simulink model "power_svc_1t_1phase_d"  (R2019a)
settings: Solver=VariableStepAuto  StartTime=0.0  StopTime=0.6  FixedStep=Ts  MaxStep=Ts  RelTol=1e-4  AbsTol=1e-4
PreLoadFcn:
  | Ts=50e-6;
libraries: powerlib x9
settings Model: ExtModeTrigMode=oneshot  ExtModeArmWhenConnect=off  ExtModeAutoUpdateStatusClock=off  Creator=MathWorks  LastModifiedBy=Thiago
settings SolverCC: AutoScaleAbsTol=off  ShapePreserveControl=EnableAll  ZeroCrossControl=EnableAll
settings DataIOCC: SaveFormat=StructureWithTime  SignalLoggingSaveFormat=ModelDataLogs  SaveOutput=off  SignalLogging=off  DSMLogging=off  SaveTime=off  ReturnWorkspaceOutputs=off  SignalLoggingName=sigsOut
settings OptimizationCC: BooleanDataType=off  ExpressionDepthLimit=2147483647  InitFltsAndDblsToZero=on  EfficientMapNaN2IntZero=off  LifeSpan=inf
settings DebuggingCC: UnderspecifiedInitializationDetection=Classic  MergeDetectMultiDrivingBlocksExec=none  CheckExecutionContextPreStartOutputMsg=on  CheckExecutionContextRuntimeOutputMsg=on  SignalResolutionControl=TryResolveAllWithWarning  MultiTaskDSMMsg=warning  MultiTaskCondExecSysMsg=none  FcnCallInpInsideContextMsg=warning  AllowSymbolicDim=off  StateNameClashWarn=warning  SFUnexpectedBacktrackingDiag=warning  SFNoUnconditionalDefaultTransitionDiag=warning  SFExecutionAtInitializationDiag=none  ArithmeticOperatorsInVariantConditions=warning
settings HardwareCC: ProdBitPerPointer=32  ProdBitPerSizeT=32  ProdBitPerPtrDiffT=32  ProdLargestAtomicFloat=None  ProdIntDivRoundTo=Undefined  ProdEndianess=Unspecified  ProdWordSize=32  ProdHWDeviceType=32-bit Generic  TargetUnknown=on
settings ModelReferenceCC: PropagateSignalLabelsOutOfModel=off
settings SFSimCC: SimUseLocalCustomCode=off
settings RTWCC: RTWUseLocalCustomCode=off
settings CodeAppCC: StateflowObjectComments=on
settings GRTTargetCC: TargetLangStandard=C89/C90 (ANSI)  CombineOutputUpdateFcns=off  GRTInterface=on
settings ConfigComp: CovMetricSettings=dw  CovSaveCumulativeToWorkspaceVar=on  CovSaveSingleToWorkspaceVar=on  CovExternalEMLEnable=off  CovSFcnEnable=off
settings SimscapeCC: SimscapeNormalizeSystem=off

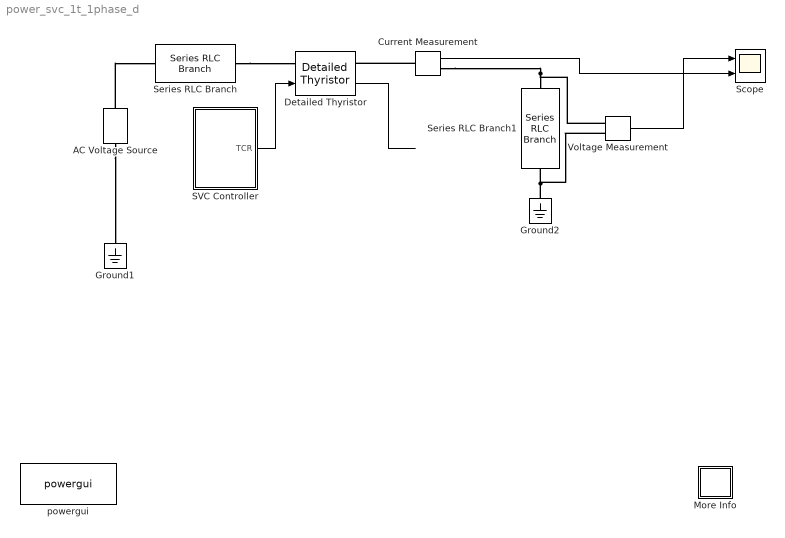
== system power_svc_1t_1phase_d ==
  AC Voltage Source : powerlib/Electrical Sources/AC Voltage Source  Amplitude=179.6  Phase=0  Frequency=60  SampleTime=0  Measurements=Voltage  BusType=swing  Pref=10e3  Qref=0  Qmin=-inf  Qmax=+inf
  Current Measurement : powerlib/Measurements/Current Measurement  PhasorSimulation=off  OutputType=Complex  PSBequivalent=0
  Detailed Thyristor : powerlib/Power Electronics/Detailed Thyristor  Ron=0.001  Lon=1e-3  Vf=0.8  IL=0.1  Tq=100e-6  IC=0.01  Rs=500  Cs=250e-9  Measurements=on
      settings: SourceProductBaseCode=PS
  Ground1 : powerlib/Elements/Ground  LConnTagsString=a
  Ground2 : powerlib/Elements/Ground  LConnTagsString=a
  More Info : Subsystem
      settings: OpenFcn=showdemo(bdroot(gcb))
      mask Display: disp('?')
  SVC Controller : Subsystem  mask(SVC Controller){OpMode=Voltage regulation, Vref=1.0, KpKi=[0 800], Xs=0.01, Bmin_max=[-1.04  3.23], Bref=2.5, Ts=Ts}
      mask prompts: OpMode "Operation mode"; Vref "Reference voltage (pu):"; KpKi "Regulator gains [ Kp  Ki ]:"; Xs "Droop (pu/100MVA):"; Bmin_max "Min. and max. primary susceptances [ Bind Bcap] (pu/100MVA):"; Bref "Susceptance Bref (pu/100MVA) (Var control mode):"; Ts "Sample time (s):"
      mask help:
      | This block implements a controller for a Static Var Compensator (SVC) consisting of one thyristor-controlled reactor bank (TCR) and three thyristor-switched capacitor banks (TSCs). Outputs TCR, TSC1, TSC2 and TSC3 are vectors of six pulses for the TCR and the three TSCs.
      | In Voltage control mode the primary voltage (Vabc_prim) is controlled at Vref within the maximum inductive and capacitive susceptance range and droop setting. In Var control mode the SVC susceptance  is  kept constant at Bref (Bref<0 for inductive mode).
      | Thyristor pulses are synchronized on secondary line-to-line voltages (Vabc_sec) of the coupling transformer, assuming a Wye/Delta (D1) connection.
      mask init:
      | Kp=KpKi(1);
      | Ki=KpKi(2);
      | Bmin=Bmin_max(1);
      | Bmax=Bmin_max(2);
      mask TypeOptions OpMode: Voltage regulation | Var control (Fixed susceptance Bref)
  Scope : Scope  NumInputPorts=2
  Series RLC Branch : powerlib/Elements/Series RLC Branch  LConnTagsString=__new0  RConnTagsString=__new0  BranchType=R  Resistance=1  Inductance=1e-6  SetiL0=on  InitialCurrent=0  Capacitance=1e-6  Setx0=off  InitialVoltage=0  Measurements=Branch voltage and current
  Series RLC Branch1 : powerlib/Elements/Series RLC Branch  LConnTagsString=__new0  RConnTagsString=__new0  BranchType=R  Resistance=10  Inductance=1e-3  SetiL0=off  InitialCurrent=0  Capacitance=1e-6  Setx0=off  InitialVoltage=0  Measurements=None
  Voltage Measurement : powerlib/Measurements/Voltage Measurement  PhasorSimulation=off  OutputType=Complex  PSBequivalent=0
  powergui : powerlib/powergui  Priority=2  SimulationMode=Continuous  SampleTime=Ts  frequency=60  Iterations=50  frequencyindice=60  Pbase=100e6  ErrMax=1e-4  UnitsV=kV  UnitsW=MW  buscounter=0  FunctionMessages=off  echomessages=off  EnableUseOfTLC=off  CurrentSourceSwitches=off  DisableSnubberDevices=off  DisableRonSwitches=off  DisableVfSwitches=off  DisplayEquations=off  AutomaticDiscreteSolvers=off  SolverType=Tustin/Backward Euler (TBE)  Interpol=off  ExternalGateDelay=off  methode=off  Ts=0  x0status=blocks  SPID=off  SwTol=0  HookPort=off  NonlinearTolerance=0  nMaxIteration=15  ContinueOnMaxIteration=off  RestoreLinks=warning  ResistiveCurrentMeasurement=off  Frange=[0:2:500]  Ylog=off  Xlog=on  ShowGrid=off  save=off  variable=ZData  structure=0  ZoomFFT=on  StartTime=0.0  cycles=1  DisplayStyle=1  fundamental=60  FreqAxis=off  MaxFrequency=1000  frequencyindicesteady=1  RmsSteady=2  display=off
  wires:
  Current Measurement/1 -> Scope/2
  Voltage Measurement/1 -> Scope/1
  Detailed Thyristor/1 -> ?
  SVC Controller/1(TCR) -> Detailed Thyristor/1
  connections:
  AC Voltage Source/LConn1 -- Ground1/LConn1
  AC Voltage Source/RConn1 -- Series RLC Branch/LConn1
  Series RLC Branch/RConn1 -- Detailed Thyristor/LConn1
  Ground2/LConn1 -- Voltage Measurement/LConn2 -- Series RLC Branch1/RConn1
  Current Measurement/LConn1 -- Detailed Thyristor/RConn1
  Current Measurement/RConn1 -- Voltage Measurement/LConn1 -- Series RLC Branch1/LConn1

== system power_svc_1t_1phase_d/More Info ==

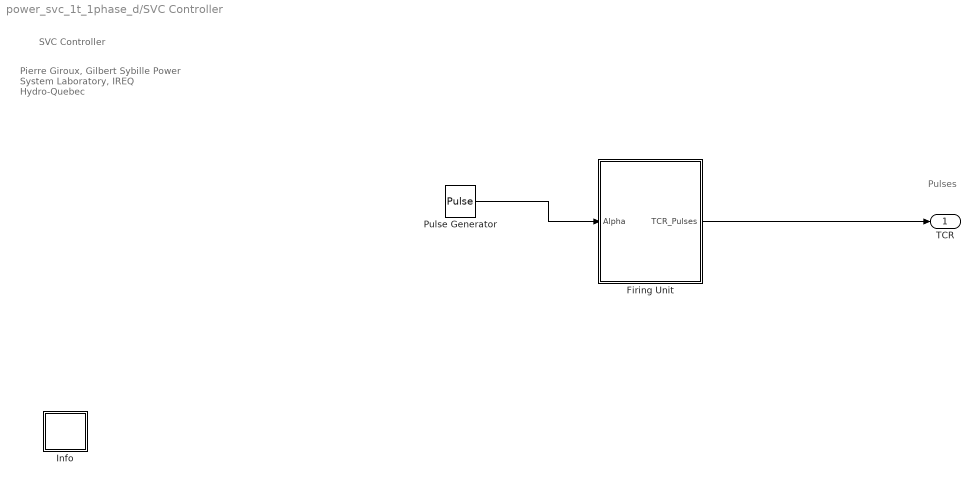
== system power_svc_1t_1phase_d/SVC Controller ==
  note: Pulses
  note: SVC Controller
  note: Pierre Giroux, Gilbert Sybille
      | Power System Laboratory, IREQ
      | Hydro-Quebec
  Firing Unit : Subsystem  mask(Firing Unit){FiringMode=Continuous, Nstep=0, ParInit=[0 60], Ts=Ts}
      mask prompts: FiringMode "Firing mode"; Nstep "Total delay (in number of time step)"; ParInit "Initial phase and frequency of input: [ Phase (degree)  Freq (Hz) ]"; Ts "Sample time:"
      mask init:
      | PhaseInit=ParInit(1);
      | FreqInit=ParInit(2);
      mask TypeOptions FiringMode: Synchronized | Continuous
  Info : Subsystem
      mask Display: disp('?')
  Pulse Generator : DiscretePulseGenerator  PulseType=Time based  Amplitude=10  Period=16.666e-3  PulseWidth=10  PhaseDelay=2.58e-3  VectorParams1D=off
  TCR : Outport
  wires:
  Firing Unit/1(TCR_Pulses) -> TCR/1
  Pulse Generator/1 -> Firing Unit/1(Alpha)

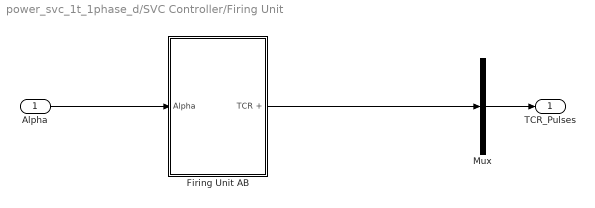
== system power_svc_1t_1phase_d/SVC Controller/Firing Unit ==
  Alpha : Inport  PortDimensions=1
  Firing Unit AB : Subsystem  mask{FiringMode=FiringMode, Nstep=Nstep, ParInit=[PhaseInit FreqInit], Ts=Ts}
      mask prompts: FiringMode "Firing Mode (1=Synchronized, 2=Continuous)"; Nstep "Total delay (in number of time step)"; ParInit "Initial phase and frequency of input: [ Phase (degree)  Freq (Hz) ]"; Ts "Sample time:"
      mask init:
      | PhaseInit=ParInit(1);
      | FreqInit=ParInit(2);
  Mux : Mux  Inputs=1
  TCR_Pulses : Outport
  wires:
  Alpha/1 -> Firing Unit AB/1(Alpha)
  Firing Unit AB/1(TCR +) -> Mux/1
  Mux/1 -> TCR_Pulses/1

== system power_svc_1t_1phase_d/SVC Controller/Info ==
  note: 1) Open-loop time constant evaluation:
  note: Xs -> Slope in pu/100MVA
      |  Ki -> Integral gain (puB/puV/s)
  note: where:
  note: Closed-loop time constant --> Tc ~= [ Xs / ( Xr + Xs ) ] * To
  note: Open-loop time constant --> To ~= 1 / ( Ki * Xs )
  note: To verify the following formula, open the loop (using the manual switch) and
      | add a 0.008 pu step to the reference voltage (Vref)
  note: 2) Misfiring simulation:
  note: To simulate a misfiring of thyristor AB+ of TSC1:
      | First switch off the TSC1 branch by adding a -0.008 pu to Vref at 0.04s
      | and then generate a firing pulse at 0.105s (one time step duration) using the Timer block

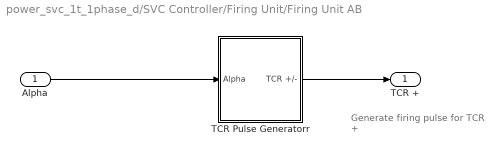
== system power_svc_1t_1phase_d/SVC Controller/Firing Unit/Firing Unit AB ==
  note: Generate firing
      | pulse for TCR +
  Alpha : Inport  PortDimensions=1
  TCR Pulse Generatorr : Subsystem  mask{Ts=Ts}
      mask prompts: Ts "Sample time:"
  TCR + : Outport
  wires:
  TCR Pulse Generatorr/1(TCR +/-) -> TCR +/1
  Alpha/1 -> TCR Pulse Generatorr/1(Alpha)

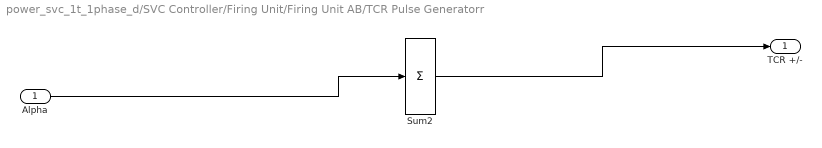
== system power_svc_1t_1phase_d/SVC Controller/Firing Unit/Firing Unit AB/TCR Pulse Generatorr ==
  Alpha : Inport  PortDimensions=1
  Sum2 : Sum  Inputs=+  SaturateOnIntegerOverflow=on  InputSameDT=on  OutDataTypeStr=Inherit: Same as first input
  TCR +/- : Outport
  wires:
  Sum2/1 -> TCR +/-/1
  Alpha/1 -> Sum2/1
